simulink model "current_feedback"  (R2023b)
settings: Solver=VariableStepAuto  StartTime=0.0  StopTime=0.001  FixedStep=0.0000009  RelTol=0.000001
libraries: cstblocks x2, simulink x1
settings Model: Creator=frenci  LastModifiedBy=frenci

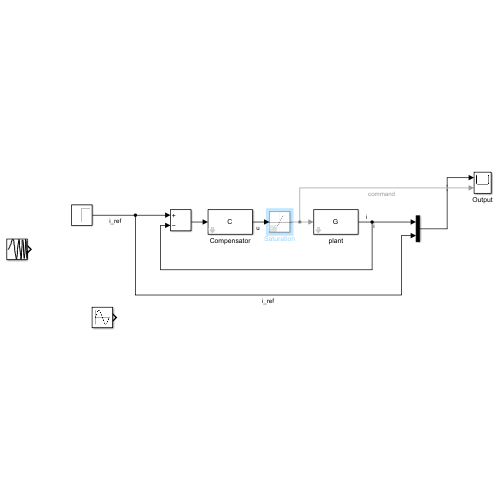
[thumbnail: Simulink's stored preview of the top-level diagram]
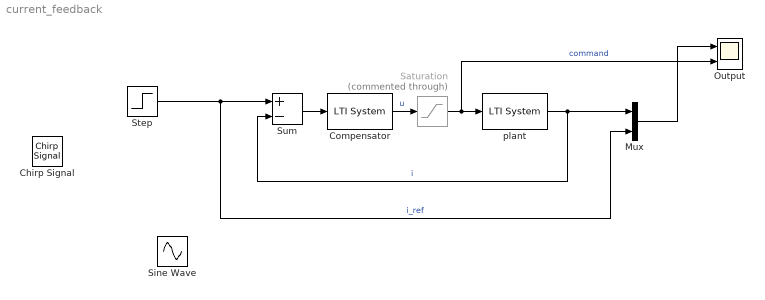
== system current_feedback ==
  Chirp Signal : simulink/Sources/Chirp Signal  f1=0  T=10  f2=1000000
  Compensator : cstblocks/LTI System  sys=C  IC=[]  PadeOrder=0
  Mux : Mux  Inputs=2
  Output : Scope  NumInputPorts=2
  Saturation : Saturate  Commented=through  UpperLimit=25  LowerLimit=-25
  Sine Wave : Sin  Amplitude=5  Frequency=2*pi*5  SampleTime=0
  Step : Step  Time=0.0001  SampleTime=0
  Sum : Sum  Inputs=+-
  plant : cstblocks/LTI System  sys=G  IC=[]  PadeOrder=0
  wires:
  Step/1 -> Mux/2, Sum/1  "i_ref"
  Sum/1 -> Compensator/1
  Compensator/1 -> Saturation/1  "u"
  plant/1 -> Sum/2, Mux/1  "i"
  Saturation/1 -> Output/2, plant/1  "command"
  Mux/1 -> Output/1
